simulink model "Final_EWASP_VC"  (R2022a)
settings: Solver=ode1  StartTime=0.0  StopTime=24*3600  FixedStep=10  RelTol=1e-3
values from neighbouring files (symbols this model uses):
  Aux_Threshold = 52    [Setup_Code_EWASP_VC.m]
  buildingAge = 2005    [Setup_Code_EWASP_VC.m]
  ceilingHeight = 2.4    [Setup_Code_EWASP_VC.m]
  conductiveHconnectMatrix = [ ... (first row only)    [Setup_Code_EWASP_VC.m]
  cRoofGreen = 100000    [Setup_Code_EWASP_VC.m]
  Defrost_After_Time = 30    [Setup_Code_EWASP_VC.m]
  DHWDemandProfile = occFreegainHotwaterElecTestPassiveOcc3(:,3)    [Setup_Code_EWASP_VC.m]
  Elec_Max = Elec_Max*(30/24.2)    [Setup_Code_EWASP_VC.m]
  Elec_Mid = Elec_Mid*(30/24.2)    [Setup_Code_EWASP_VC.m]
  Elec_Min = Elec_Min*(30/24.2)    [Setup_Code_EWASP_VC.m]
  ElecDemandProfile = occFreegainHotwaterElecTestPassiveOcc3(:,4)    [Setup_Code_EWASP_VC.m]
  ElecFixed = [Elec_Max(6,2) Elec_Max(6,4) Elec_Max(6,6) Elec_Max(6,7) ... (first row only)    [Setup_Code_EWASP_VC.m]
  floorOrCeilingArea = floorOrCeilingArea*1.15    [Setup_Code_EWASP_VC.m]
  forceCold = 0    [Setup_Code_EWASP_VC.m]
  freegain = occFreegainHotwaterElecTestPassiveOcc3(:,2)-max(occupancy)*25    [Setup_Code_EWASP_VC.m]
  furnitureModelOn = 1    [Setup_Code_EWASP_VC.m]
  Heat_Max = Heat_Max*(30/24.2)    [Setup_Code_EWASP_VC.m]
  Heat_Mid = Heat_Mid*(30/24.2)    [Setup_Code_EWASP_VC.m]
  Heat_Min = Heat_Min*(30/24.2)    [Setup_Code_EWASP_VC.m]
  HeatFixed = [Heat_Max(6,2) Heat_Max(6,4) Heat_Max(6,6) Heat_Max(6,7) ... (first row only)    [Setup_Code_EWASP_VC.m]
  HeatingOnProfile = repmat(HeatingOnProfile,365,1)    [Setup_Code_EWASP_VC.m]
  HEX_ReturnLowerLimit = 52.5    [Setup_Code_EWASP_VC.m]
  HEX_ReturnUpperLimit = 55    [Setup_Code_EWASP_VC.m]
  LeakMultiplier = 1+(2*(rand()-0.5)/10)    [Setup_Code_EWASP_VC.m]
  loopCap = 15    [Setup_Code_EWASP_VC.m]
  maxOcc = max(occupancyProfile)    [Setup_Code_EWASP_VC.m]
  NESW_wallArea = max(NESW_Lengths*ceilingHeight-NESW_Windows,0)    [Setup_Code_EWASP_VC.m]
  NESW_Windows = [ ... (first row only)    [Setup_Code_EWASP_VC.m]
  numRooms = roomCount    [Setup_Code_EWASP_VC.m]
  offsetDays = 0    [Setup_Code_EWASP_VC.m]
  pumpChoice = pumpChoices(MinIndex,1)    [Setup_Code_EWASP_VC.m]
  pumpRamp = 180    [Setup_Code_EWASP_VC.m]
  ReturnLowerLimit = 37.5    [Setup_Code_EWASP_VC.m]
  ReturnUpperLimit = 40    [Setup_Code_EWASP_VC.m]
  RoofIrradiance = Flat_NS_EW_RoofIrradiance(:,1)    [Setup_Code_EWASP_VC.m]
  roofStartTemp = ones(11,1)*20    [Setup_Code_EWASP_VC.m]
  rooftype = 0    [Setup_Code_EWASP_VC.m]
  RoomDataMatrix = [zeros(1,12);ones(1,12)*wallDensity;zeros(1,12);ones(1,12)*wallU;ones(1,12)*windowU;ones(1,12)*floorU;ones(1,12)*ceilingU;zeros(1,12);windowArea, 0;floorOrCeilingArea;zeros(1,12);floorOrCeilingArea*ceilingHeight]    [Setup_Code_EWASP_VC.m]
  roomVol = roomVol*1.15    [Setup_Code_EWASP_VC.m]
  slabStartTemp = (GroundTempTimeSeries(offsetDays*1440+1,1)+thermostatSetting)/2    [Setup_Code_EWASP_VC.m]
  SlackRequest = zeros(1440,1)    [Setup_Code_EWASP_VC.m]
  SolarThermalExists = 0    [Setup_Code_EWASP_VC.m]
  SourceFixed = HeatFixed-ElecFixed    [Setup_Code_EWASP_VC.m]
  StateSeries = StateSeriesGenerator(22,7,1)    [Setup_Code_EWASP_VC.m]
  Tank_Lower_Temp = 49.5    [Setup_Code_EWASP_VC.m]
  Tank_Upper_Temp = 52    [Setup_Code_EWASP_VC.m]
  Tank_Volume_m3 = 0.15    [Setup_Code_EWASP_VC.m]
  TankHeatHour = randi([1 5])-1    [Setup_Code_EWASP_VC.m]
  thermostatSetting = 20.0    (= 20)    [Setup_Code_EWASP_VC.m]
  upDown = [0;0;0;0;1;1;1;1;1;1;1]    [Setup_Code_EWASP_VC.m]
  variableASHP = 1    [Setup_Code_EWASP_VC.m]
  wallStartTempExt = thermostatSetting*(0.266+0.00215*outdoorStartTemp+0.018*wallU+0.00113*outdoorStartTemp*wallU+0.0068*wallU^2)    [Setup_Code_EWASP_VC.m]
undefined symbols (not defined in the file or in its folder): a, ceilingU, condUDMatrix, convUDMatrix, deltaPEXPANDED_E, deltaPEXPANDED_E2, deltaPEXPANDED_N, deltaPEXPANDED_N2, deltaPEXPANDED_S, deltaPEXPANDED_S2, deltaPEXPANDED_W, deltaPEXPANDED_W2, DesiredDHWTemp, DesiredFlowTempVsInOutDeltaTemp, DiffuseHorizontal, DiscIntNeverNeededParam, DNI, dwnAndConcrete, DWORK_A_HX, DWORK_CHK_FLU, DWORK_CP_NODE, DWORK_DH, DWORK_FLUID, DWORK_HCON, DWORK_LOSS, DWORK_MDOTDOWN, DWORK_MDOTIN, DWORK_MDOTUP, DWORK_MIX, DWORK_PRESS, DWORK_QDOTIN, DWORK_RHO_NODE, DWORK_TIN, DWORK_TS_OLD, DWORK_V_NODE, GroundTempTimeSeries, HCM, HCM2, HCM_closed, HCM_closed2, intermediateU, IsTop, massFlowMatrix, neighbourMatrix, numericalRoomUse, RadiatorMatrix, room2roomflowmatrix_E, room2roomflowmatrix_E2, room2roomflowmatrix_N, room2roomflowmatrix_N2, room2roomflowmatrix_S, room2roomflowmatrix_S2, room2roomflowmatrix_W, room2roomflowmatrix_W2, StateAirInEXPANDED_E, StateAirInEXPANDED_E2, StateAirInEXPANDED_N, StateAirInEXPANDED_N2, StateAirInEXPANDED_S, StateAirInEXPANDED_S2 ... (+23)
libraries: simulink x6, dspsigops x4, dspmtrx3 x4, carnot x3, spsEdgeDetectorLib x2, dspstat3 x2, powerlib_meascontrol x1, simulink_extras x1
(part 27 of 27)

== matlab function Final_EWASP_VC/Subsystem_Room8/Bedroom3/Subsystem4/MATLAB Function2 ==
  data: Angle_NEWS output; angleSeries input; NEWS_DNI output; DNISeries input; DiffSeries input; Time input; offsetDays input; NESW_Windows input; roomNumber input; NEWS_Diff output
function [Angle_NEWS,NEWS_DNI,NEWS_Diff] = SolarSeriesDataExtractor(angleSeries,DNISeries,DiffSeries,Time,offsetDays,NESW_Windows,roomNumber)

%deltaTexternalNEWS=zeros(1,4);

Angle_NEWS=angleSeries(ceil((offsetDays*1440)+Time/60+0.00001),1:4);
DNI=DNISeries(ceil((offsetDays*1440)+Time/60+0.00001),1);
Diff=DiffSeries(ceil((offsetDays*1440)+Time/60+0.00001),1);%extracts correct Diff per unit horizontal area for the timestep (corrected for wall tilt at a later stage

NEWS_windowArea=NESW_Windows;
NEWS_windowArea([3 4],:)=NEWS_windowArea([4 3],:);

RoomWindowAreas_NEWS=NEWS_windowArea(:,roomNumber)';


NEWS_DNI=RoomWindowAreas_NEWS*DNI;
NEWS_Diff=RoomWindowAreas_NEWS*Diff;

== matlab function Final_EWASP_VC/Subsystem_Room2/Kitchen/Subsystem1/MATLAB Function1 ==
  data: PU_AreaIrradianceTotal output; angleSeries input; NEWS_Irradiance output; DNISeries input; DiffSeries input; Time input; offsetDays input; SurfaceAlbedo input; NESW_wallArea input; roomNumber input; c_OutPU input; deltaTexternalNEWS output
function [PU_AreaIrradianceTotal, NEWS_Irradiance,deltaTexternalNEWS] = SolarSeriesToExtWallGains(angleSeries,DNISeries,DiffSeries,Time,offsetDays,SurfaceAlbedo,NESW_wallArea,roomNumber,c_OutPU)

%deltaTexternalNEWS=zeros(1,4);

Angle_NEWS=angleSeries(ceil((offsetDays*1440)+Time/60+0.00001),1:4);
DNI=DNISeries(ceil((offsetDays*1440)+Time/60+0.00001),1);

PU_AreaDiff=DiffSeries(ceil((offsetDays*1440)+Time/60+0.00001),1)/2;%extracts correct Diff for the timestep, factor of 1/2 corrects for 90 degree walls (so only half Diff irradiance can be utilised)
PU_AreaDNI=cos(deg2rad(Angle_NEWS))*DNI;
NEWS_wallArea=NESW_wallArea;
NEWS_wallArea([3 4],:)=NEWS_wallArea([4 3],:);

RoomWallAreas_NEWS=NEWS_wallArea(:,roomNumber)';
PU_AreaIrradianceTotal=(PU_AreaDNI+PU_AreaDiff)*(1-SurfaceAlbedo);

NEWS_Irradiance=RoomWallAreas_NEWS.*PU_AreaIrradianceTotal;
deltaTexternalNEWS=NEWS_Irradiance./(c_OutPU*RoomWallAreas_NEWS);

for i=1:4
   
    if RoomWallAreas_NEWS(1,i)==0
        deltaTexternalNEWS(1,i)=0;
    else
        
    end
    
end

== matlab function Final_EWASP_VC/Subsystem_Room5/Landing/Subsystem2/MATLAB Function1 ==
  data: PU_AreaIrradianceTotal output; angleSeries input; NEWS_Irradiance output; DNISeries input; DiffSeries input; Time input; offsetDays input; SurfaceAlbedo input; NESW_wallArea input; roomNumber input; c_OutPU input; deltaTexternalNEWS output
function [PU_AreaIrradianceTotal, NEWS_Irradiance,deltaTexternalNEWS] = SolarSeriesToExtWallGains(angleSeries,DNISeries,DiffSeries,Time,offsetDays,SurfaceAlbedo,NESW_wallArea,roomNumber,c_OutPU)

%deltaTexternalNEWS=zeros(1,4);

Angle_NEWS=angleSeries(ceil((offsetDays*1440)+Time/60+0.00001),1:4);
DNI=DNISeries(ceil((offsetDays*1440)+Time/60+0.00001),1);

PU_AreaDiff=DiffSeries(ceil((offsetDays*1440)+Time/60+0.00001),1)/2;%extracts correct Diff for the timestep, factor of 1/2 corrects for 90 degree walls (so only half Diff irradiance can be utilised)
PU_AreaDNI=cos(deg2rad(Angle_NEWS))*DNI;
NEWS_wallArea=NESW_wallArea;
NEWS_wallArea([3 4],:)=NEWS_wallArea([4 3],:);

RoomWallAreas_NEWS=NEWS_wallArea(:,roomNumber)';
PU_AreaIrradianceTotal=(PU_AreaDNI+PU_AreaDiff)*(1-SurfaceAlbedo);

NEWS_Irradiance=RoomWallAreas_NEWS.*PU_AreaIrradianceTotal;
deltaTexternalNEWS=NEWS_Irradiance./(c_OutPU*RoomWallAreas_NEWS);

for i=1:4
   
    if RoomWallAreas_NEWS(1,i)==0
        deltaTexternalNEWS(1,i)=0;
    else
        
    end
    
end

== matlab function Final_EWASP_VC/Subsystem_Room1/Lounge//Dining/Radiator w//Thermostatic Control2/MATLAB Function ==
  data: MassRad input; heatCapRad input; mdotRad input; Tflow input; Tnode1 input; Tnode2 input; deltaT1 output; deltaT2 output; nominalHeat input; nominalDeltaT input; Troom input; Qtoroom output
function [deltaT1,deltaT2,Qtoroom]=fcn(MassRad,heatCapRad, mdotRad, Tflow,Tnode1,Tnode2,nominalHeat,nominalDeltaT,Troom)


if  Tnode1 == Tnode2 || Tnode1 <= Troom || Tnode2 <= Troom %if lmtd methodnis problemtatic, use arithmetic method
    radiatorHeatOut=sign(((Tnode1+Tnode2) /2)-Troom)*abs((nominalHeat)*((((Tnode1+Tnode2) /2)-Troom)/nominalDeltaT)^1.3);
deltaT1=(mdotRad*4180*(Tflow-Tnode1))/((heatCapRad*MassRad)/2);
deltaT2=(mdotRad*4180*(Tnode1-Tnode2)-radiatorHeatOut)/((heatCapRad*MassRad)/2);

else 
  
   radiatorHeatOut=(nominalHeat/nominalDeltaT^1.3)*((Tnode1-Tnode2)/log((Tnode1-Troom)/(Tnode2-Troom)))^1.3;
   radiatorHeatOut=real(radiatorHeatOut);
deltaT1=(mdotRad*4180*(Tflow-Tnode1))/((heatCapRad*MassRad)/2);
deltaT2=(mdotRad*4180*(Tnode1-Tnode2)-radiatorHeatOut)/((heatCapRad*MassRad)/2);

   deltaT1=real(deltaT1);
   deltaT2=real(deltaT2);
    

end

Qtoroom=real(radiatorHeatOut);

== matlab function Final_EWASP_VC/Airflow Model/MATLAB Function ==
  data: WindSpeed input; WindIndex output; Tin_Avg input; T_out input; StackIndex output; WindDir input; DirIndex output
function [WindIndex,StackIndex,DirIndex] = fcn(WindSpeed,Tin_Avg,T_out,WindDir)

WindspeedLookUp=[0,1,2,3,5,8,12,15,18,21,25,30];
DeltaTemp=[0, 10, 20];

delT=(Tin_Avg-T_out);


[~,closestIndex] = min(abs(WindspeedLookUp-WindSpeed));
[~,closestIndex2] = min(abs(DeltaTemp-delT));

if WindDir == 1
    DirIndex=1;
elseif WindDir == 2
DirIndex=2;
elseif WindDir == 3
DirIndex=3;
elseif WindDir == 4
    DirIndex=4;
else
    error('wind direction must be either 1 (north) 2 (east) 3 (south) or 4 (west)')
end
WindIndex = closestIndex;
StackIndex = closestIndex2;

== matlab function Final_EWASP_VC/Airflow Model/MATLAB Function1 ==
  settings: updateMethod=DISCRETE  sampleTime=900
  data: WindSpeed input; WindIndex output; Tin_Avg input; T_out input; StackIndex output; WindDir input; DirIndex output
function [WindIndex,StackIndex,DirIndex] = fcn(WindSpeed,Tin_Avg,T_out,WindDir)

WindspeedLookUp=[0,1,2,3,5,8,12,15,18,21,25,30];
DeltaTemp=[0, 10, 20];

delT=(Tin_Avg-T_out);


[~,closestIndex] = min(abs(WindspeedLookUp-WindSpeed));
[~,closestIndex2] = min(abs(DeltaTemp-delT));

if WindDir == 1
    DirIndex=1;
elseif WindDir == 2
DirIndex=2;
elseif WindDir == 3
DirIndex=3;
elseif WindDir == 4
    DirIndex=4;
else
    error('wind direction must be either 1 (north) 2 (east) 3 (south) or 4 (west)')
end
WindIndex = closestIndex;
StackIndex = closestIndex2;

== matlab function Final_EWASP_VC/Airflow Model/StateLoader ==
  settings: updateMethod=DISCRETE  sampleTime=10
  data: R2R_out output size=[11 11]; windIndex input; stackIndex input; windDir input; room2roomflowmatrix_N input; room2roomflowmatrix_E input; room2roomflowmatrix_S input; room2roomflowmatrix_W input; StateAirInEXPANDED_N input; StateAirInEXPANDED_E input; StateAirInEXPANDED_S input; StateAirInEXPANDED_W input; StateAirOutEXPANDED_N input; StateAirOutEXPANDED_E input; StateAirOutEXPANDED_S input; StateAirOutEXPANDED_W input; deltaPEXPANDED_N input; deltaPEXPANDED_E input; deltaPEXPANDED_S input; deltaPEXPANDED_W input; numRooms input; StateAirIn_out output size=[11 1]; StateAirOut_out output size=[11 1]; deltaP output
function [R2R_out, StateAirIn_out,StateAirOut_out,deltaP] = fcn(windIndex,stackIndex,windDir,room2roomflowmatrix_N,room2roomflowmatrix_E,room2roomflowmatrix_S,room2roomflowmatrix_W,StateAirInEXPANDED_N,StateAirInEXPANDED_E,StateAirInEXPANDED_S,StateAirInEXPANDED_W,StateAirOutEXPANDED_N,StateAirOutEXPANDED_E,StateAirOutEXPANDED_S,StateAirOutEXPANDED_W,deltaPEXPANDED_N,deltaPEXPANDED_E,deltaPEXPANDED_S,deltaPEXPANDED_W,numRooms)

if windDir == 1
    
R2R_out=room2roomflowmatrix_N((windIndex-1)*numRooms+1:windIndex*numRooms,(stackIndex-1)*numRooms+1:stackIndex*numRooms);
StateAirIn_out=StateAirInEXPANDED_N((windIndex-1)*numRooms+1:windIndex*numRooms,stackIndex);
StateAirOut_out=StateAirOutEXPANDED_N((windIndex-1)*numRooms+1:windIndex*numRooms,stackIndex);
deltaP=deltaPEXPANDED_N(windIndex,stackIndex);

elseif windDir == 2
    
    R2R_out=room2roomflowmatrix_E((windIndex-1)*numRooms+1:windIndex*numRooms,(stackIndex-1)*numRooms+1:stackIndex*numRooms);
StateAirIn_out=StateAirInEXPANDED_E((windIndex-1)*numRooms+1:windIndex*numRooms,stackIndex);
StateAirOut_out=StateAirOutEXPANDED_E((windIndex-1)*numRooms+1:windIndex*numRooms,stackIndex);
deltaP=deltaPEXPANDED_E(windIndex,stackIndex);
    
elseif windDir == 3
        
    R2R_out=room2roomflowmatrix_S((windIndex-1)*numRooms+1:windIndex*numRooms,(stackIndex-1)*numRooms+1:stackIndex*numRooms);
StateAirIn_out=StateAirInEXPANDED_S((windIndex-1)*numRooms+1:windIndex*numRooms,stackIndex);
StateAirOut_out=StateAirOutEXPANDED_S((windIndex-1)*numRooms+1:windIndex*numRooms,stackIndex);
deltaP=deltaPEXPANDED_S(windIndex,stackIndex);
    
elseif windDir == 4
            
    R2R_out=room2roomflowmatrix_W((windIndex-1)*numRooms+1:windIndex*numRooms,(stackIndex-1)*numRooms+1:stackIndex*numRooms);
StateAirIn_out=StateAirInEXPANDED_W((windIndex-1)*numRooms+1:windIndex*numRooms,stackIndex);
StateAirOut_out=StateAirOutEXPANDED_W((windIndex-1)*numRooms+1:windIndex*numRooms,stackIndex);
deltaP=deltaPEXPANDED_W(windIndex,stackIndex);
    
else
  error('windDir must equal 1,2,3, or 4')          
end

%R2R_out=R2R_out+zeros(11,11);
%R2R_out=R2R_out(11,11);
%StateAirIn_out=StateAirIn_out+zeros(11,1);
%StateAirOut_out=StateAirOut_out+zeros(11,1);

== matlab function Final_EWASP_VC/Airflow Model/StateLoader1 ==
  settings: updateMethod=DISCRETE  sampleTime=10
  data: windIndex input; stackIndex input; windDir input; room2roomflowmatrix_N input; room2roomflowmatrix_E input; room2roomflowmatrix_S input; room2roomflowmatrix_W input; StateAirInEXPANDED_N input; StateAirInEXPANDED_E input; StateAirInEXPANDED_S input; StateAirInEXPANDED_W input; StateAirOutEXPANDED_N input; StateAirOutEXPANDED_E input; StateAirOutEXPANDED_S input; StateAirOutEXPANDED_W input; deltaPEXPANDED_N input; deltaPEXPANDED_E input; deltaPEXPANDED_S input; deltaPEXPANDED_W input; numRooms input; R2R_out output size=[11 11]; StateAirIn_out output size=[11 1]; StateAirOut_out output size=[11 1]; deltaP output
function [R2R_out,StateAirIn_out,StateAirOut_out,deltaP] = fcn(windIndex,stackIndex,windDir,room2roomflowmatrix_N,room2roomflowmatrix_E,room2roomflowmatrix_S,room2roomflowmatrix_W,StateAirInEXPANDED_N,StateAirInEXPANDED_E,StateAirInEXPANDED_S,StateAirInEXPANDED_W,StateAirOutEXPANDED_N,StateAirOutEXPANDED_E,StateAirOutEXPANDED_S,StateAirOutEXPANDED_W,deltaPEXPANDED_N,deltaPEXPANDED_E,deltaPEXPANDED_S,deltaPEXPANDED_W,numRooms)

if windDir == 1
    
R2R_out=room2roomflowmatrix_N((windIndex-1)*numRooms+1:windIndex*numRooms,(stackIndex-1)*numRooms+1:stackIndex*numRooms);
StateAirIn_out=StateAirInEXPANDED_N((windIndex-1)*numRooms+1:windIndex*numRooms,stackIndex);
StateAirOut_out=StateAirOutEXPANDED_N((windIndex-1)*numRooms+1:windIndex*numRooms,stackIndex);
deltaP=deltaPEXPANDED_N(windIndex,stackIndex);

elseif windDir == 2
    
    R2R_out=room2roomflowmatrix_E((windIndex-1)*numRooms+1:windIndex*numRooms,(stackIndex-1)*numRooms+1:stackIndex*numRooms);
StateAirIn_out=StateAirInEXPANDED_E((windIndex-1)*numRooms+1:windIndex*numRooms,stackIndex);
StateAirOut_out=StateAirOutEXPANDED_E((windIndex-1)*numRooms+1:windIndex*numRooms,stackIndex);
deltaP=deltaPEXPANDED_E(windIndex,stackIndex);
    
elseif windDir == 3
        
    R2R_out=room2roomflowmatrix_S((windIndex-1)*numRooms+1:windIndex*numRooms,(stackIndex-1)*numRooms+1:stackIndex*numRooms);
StateAirIn_out=StateAirInEXPANDED_S((windIndex-1)*numRooms+1:windIndex*numRooms,stackIndex);
StateAirOut_out=StateAirOutEXPANDED_S((windIndex-1)*numRooms+1:windIndex*numRooms,stackIndex);
deltaP=deltaPEXPANDED_S(windIndex,stackIndex);
    
elseif windDir == 4
            
    R2R_out=room2roomflowmatrix_W((windIndex-1)*numRooms+1:windIndex*numRooms,(stackIndex-1)*numRooms+1:stackIndex*numRooms);
StateAirIn_out=StateAirInEXPANDED_W((windIndex-1)*numRooms+1:windIndex*numRooms,stackIndex);
StateAirOut_out=StateAirOutEXPANDED_W((windIndex-1)*numRooms+1:windIndex*numRooms,stackIndex);
deltaP=deltaPEXPANDED_W(windIndex,stackIndex);
    
else
  error('windDir must equal 1,2,3, or 4')          
end

%R2R_out=R2R_out+zeros(11,11);
%StateAirIn_out=StateAirIn_out+zeros(11,1);
%StateAirOut_out=StateAirOut_out+zeros(11,1);

== matlab function Final_EWASP_VC/Airflow Model/Subsystem1/Subsystem/Actual buoyancy ==
  data: u input; y output; v input; w input
function y  = fcn(u,v,w)

y = w.*(1-u./v);

== matlab function Final_EWASP_VC/Airflow Model/Subsystem1/Subsystem/Remove nan values ==
  data: y output; u input
function y  = fcn(u)

u(isnan(u))=0;
y=u;

== matlab function Final_EWASP_VC/Airflow Model/Subsystem1/Subsystem/Subsystem1/Temp2density ==
  data: u input; y output
function y  = fcn(u)

y = -0.0042*u+1.2898;

== matlab function Final_EWASP_VC/Airflow Model/Subsystem1/Subsystem/Subsystem1/Temp2density1 ==
  data: u input; y output
function y  = fcn(u)

y = -0.0042*u+1.2898;

== matlab function Final_EWASP_VC/Airflow Model/Subsystem1/Subsystem/Subsystem1/Temp2density2 ==
  data: u input; y output
function y  = fcn(u)

y = -0.0042*u+1.2898;

== matlab function Final_EWASP_VC/Airflow Model/Subsystem1/Subsystem/Subsystem1/floorDensityCorrection ==
  data: u input; y output; v input; w input
function y  = fcn(u,v,w)

a=u-u.*2.718^((-9.80665*0.0289644*2.7)/(8.31446*(w+273.15)));


y=repmat(v,1,length(v))*a;

== matlab function Final_EWASP_VC/Airflow Model/Subsystem1/Subsystem/Subsystem1/tempVector to average ==
  data: u input; y output
function y = fcn(u)

y = mean(u);

== matlab function Final_EWASP_VC/Subsystem_Room1/Lounge//Dining/Subsystem1/MATLAB Function ==
  data: uValWall input; deltaTint output; c_InPU input; c_MidPU input; c_OutPU input; T_InWallNEWS input; T_MidWallNEWS input; T_OutWallNEWS input; T_Room input; T_AmbientSeries input; windSpeedSeries input; deltaTmid output; deltaTout output; NESW_wallArea input; roomNumber input; logRoomHeatLoss output; Time input; offsetDays input
function [deltaTint,deltaTmid,deltaTout,logRoomHeatLoss] = fcn(uValWall,c_InPU,c_MidPU,c_OutPU,T_InWallNEWS, T_MidWallNEWS,T_OutWallNEWS,T_Room,T_AmbientSeries,windSpeedSeries,NESW_wallArea,roomNumber,Time,offsetDays)




  deltaTint=zeros(1,4);
   deltaTmid=zeros(1,4);
    deltaTout=zeros(1,4);
    logRoomHeatLoss=zeros(1,4);

    v_Wind=windSpeedSeries(ceil((offsetDays*1440)+Time/60+0.00001),1);
   T_Ambient=T_AmbientSeries(ceil((offsetDays*1440)+Time/60+0.00001),1);
    
k_InMid=uValWall*2;
k_OutMid=uValWall*2;


NEWS_wallArea=NESW_wallArea;
NEWS_wallArea([3 4],:)=NEWS_wallArea([4 3],:);
RoomWallAreas_NEWS=NEWS_wallArea(:,roomNumber)';


for i=1:4
    
    if RoomWallAreas_NEWS(1,i)>0

c_In=c_InPU*RoomWallAreas_NEWS(1,i);
c_Mid=c_MidPU*RoomWallAreas_NEWS(1,i);
c_Out=c_OutPU*RoomWallAreas_NEWS(1,i);

T_InWall=T_InWallNEWS(1,i);
T_MidWall=T_MidWallNEWS(1,i);
T_OutWall=T_OutWallNEWS(1,i);
    
aA=[-(k_InMid*RoomWallAreas_NEWS(1,i))/c_In (k_InMid*RoomWallAreas_NEWS(1,i))/c_In 0
 (k_InMid*RoomWallAreas_NEWS(1,i))/c_Mid -((k_InMid+k_OutMid)*RoomWallAreas_NEWS(1,i))/c_Mid (k_OutMid*RoomWallAreas_NEWS(1,i))/c_Mid
 0 (k_OutMid*RoomWallAreas_NEWS(1,i))/c_Out -(k_OutMid*RoomWallAreas_NEWS(1,i))/c_Out];

bA=[1/c_In 0 0
 0 1/c_Mid 0
 0 0 1/c_Out];
    
ab=[T_InWall
    T_MidWall
    T_OutWall];

bb=[(2.5*(T_Room-T_InWall)+5.6*(T_Room-T_InWall))*RoomWallAreas_NEWS(1,i)
0    
(2.8+3*v_Wind)*(T_Ambient-T_OutWall)+5.6*(T_Ambient-T_OutWall)*RoomWallAreas_NEWS(1,i)];

deltaT=aA*ab+bA*bb;

    deltaTint(1,i)=deltaT(1,1);
   deltaTmid(1,i)=deltaT(2,1);
    deltaTout(1,i)=deltaT(3,1);
    
    logRoomHeatLoss(1,i)=bb(1,1);
    
    else
        
        deltaTint(1,i)=0;
   deltaTmid(1,i)=0;
    deltaTout(1,i)=0;
        
    logRoomHeatLoss(1,i)=0;
    
    end
    
end

== matlab function Final_EWASP_VC/Airflow Model/Subsystem1/Subsystem/Subsystem1/tempVector to matrices ==
  data: u input; y output; x output
function [y,x] = fcn(u)

y = repmat(u,1,size(u,1));
x=y';

== matlab function Final_EWASP_VC/Airflow Model/Subsystem1/Subsystem/max buoyancy ==
  data: u input; y output; v input
function y  = fcn(u,v)

y = (u*0.055).*abs(9.81*v.*ones(size(u,1),size(u,1))./u).^0.5;

== matlab function Final_EWASP_VC/Airflow Model/Subsystem1/Subsystem/pflood ==
  data: u input; y output
function y  = fcn(u)

y = ((1/0.3)*0.942^2*9.81*u*1)/(2*1);

== matlab function Final_EWASP_VC/Airflow Model/Subsystem1/Subsystem/tempVector to matrices ==
  data: u input; y output; x output
function [y,x] = fcn(u)

a=u;
y = repmat(a,1,length(a));
x=y';

== matlab function Final_EWASP_VC/Airflow Model/Subsystem2/Subsystem/Actual buoyancy ==
  data: u input; y output; v input; w input
function y  = fcn(u,v,w)

y = w.*(1-u./v);

== matlab function Final_EWASP_VC/Airflow Model/Subsystem2/Subsystem/Remove nan values ==
  data: y output; u input
function y  = fcn(u)

u(isnan(u))=0;
y=u;

== matlab function Final_EWASP_VC/Airflow Model/Subsystem2/Subsystem/Subsystem1/Temp2density ==
  data: u input; y output
function y  = fcn(u)

y = -0.0042*u+1.2898;

== matlab function Final_EWASP_VC/Airflow Model/Subsystem2/Subsystem/Subsystem1/Temp2density1 ==
  data: u input; y output
function y  = fcn(u)

y = -0.0042*u+1.2898;

== matlab function Final_EWASP_VC/Airflow Model/Subsystem2/Subsystem/Subsystem1/Temp2density2 ==
  data: u input; y output
function y  = fcn(u)

y = -0.0042*u+1.2898;

== matlab function Final_EWASP_VC/Airflow Model/Subsystem2/Subsystem/Subsystem1/floorDensityCorrection ==
  data: u input; y output; v input; w input
function y  = fcn(u,v,w)

a=u-u.*2.718^((-9.80665*0.0289644*2.7)/(8.31446*(w+273.15)));


y=repmat(v,1,length(v))*a;

== matlab function Final_EWASP_VC/Airflow Model/Subsystem2/Subsystem/Subsystem1/tempVector to average ==
  data: u input; y output
function y = fcn(u)

y = mean(u);

== matlab function Final_EWASP_VC/Airflow Model/Subsystem2/Subsystem/Subsystem1/tempVector to matrices ==
  data: u input; y output; x output
function [y,x] = fcn(u)

y = repmat(u,1,size(u,1));
x=y';

== matlab function Final_EWASP_VC/Airflow Model/Subsystem2/Subsystem/max buoyancy ==
  data: u input; y output; v input
function y  = fcn(u,v)

y = (u*0.055).*abs(9.81*v.*ones(size(u,1),size(u,1))./u).^0.5;

== matlab function Final_EWASP_VC/Airflow Model/Subsystem2/Subsystem/pflood ==
  data: u input; y output
function y  = fcn(u)

y = ((1/0.3)*0.942^2*9.81*u*1)/(2*1);

== matlab function Final_EWASP_VC/Airflow Model/Subsystem2/Subsystem/tempVector to matrices ==
  data: u input; y output; x output
function [y,x] = fcn(u)

a=u;
y = repmat(a,1,length(a));
x=y';

== matlab function Final_EWASP_VC/Subsystem_Room1/Lounge//Dining/Subsystem3/MATLAB Function ==
  data: uValWall input; deltaTint output; c_InPU input; c_MidPU input; c_OutPU input; T_InWall input; T_MidWall input; T_OutWall input; T_Room input; T_AmbientSeries input; windSpeedSeries input; deltaTmid output; deltaTout output; ceilArea input; roomNumber input; logRoomHeatLoss output; Time input; offsetDays input
function [deltaTint,deltaTmid,deltaTout,logRoomHeatLoss] = fcn(uValWall,c_InPU,c_MidPU,c_OutPU,T_InWall, T_MidWall,T_OutWall,T_Room,T_AmbientSeries,windSpeedSeries,ceilArea,roomNumber,Time,offsetDays)




  deltaTint=zeros(1,1);
   deltaTmid=zeros(1,1);
    deltaTout=zeros(1,1);
    logRoomHeatLoss=zeros(1,1);

    v_Wind=windSpeedSeries(ceil((offsetDays*1440)+Time/60+0.00001),1);
   T_Ambient=T_AmbientSeries(ceil((offsetDays*1440)+Time/60+0.00001),1);
    
k_InMid=uValWall*2;
k_OutMid=uValWall*2;




    
    if ceilArea>0

c_In=c_InPU*ceilArea;
c_Mid=c_MidPU*ceilArea;
c_Out=c_OutPU*ceilArea;

    
aA=[-(k_InMid*ceilArea)/c_In (k_InMid*ceilArea)/c_In 0
 (k_InMid*ceilArea)/c_Mid -((k_InMid+k_OutMid)*ceilArea)/c_Mid (k_OutMid*ceilArea)/c_Mid
 0 (k_OutMid*ceilArea)/c_Out -(k_OutMid*ceilArea)/c_Out];

bA=[1/c_In 0 0
 0 1/c_Mid 0
 0 0 1/c_Out];
    
ab=[T_InWall
    T_MidWall
    T_OutWall];

bb=[(2.5*(T_Room-T_InWall)+5.6*(T_Room-T_InWall))*ceilArea
0    
(2.8+3*v_Wind)*(T_Ambient-T_OutWall)+5.6*(T_Ambient-T_OutWall)*ceilArea];

deltaT=aA*ab+bA*bb;

    deltaTint=deltaT(1,1);
   deltaTmid=deltaT(2,1);
    deltaTout=deltaT(3,1);
    
    logRoomHeatLoss=bb(1,1);
    
    else
        
        deltaTint=0;
   deltaTmid=0;
    deltaTout=0;
        
    logRoomHeatLoss=0;
    
    end

== matlab function Final_EWASP_VC/Subsystem_Room7/Bedroom 2/Subsystem3/MATLAB Function ==
  data: uValWall input; deltaTint output; c_InPU input; c_MidPU input; c_OutPU input; T_InWallNEWS input; T_MidWallNEWS input; T_OutWallNEWS input; T_Room input; T_AmbientSeries input; windSpeedSeries input; deltaTmid output; deltaTout output; NESW_wallArea input; roomNumber input; logRoomHeatLoss output; Time input; offsetDays input
function [deltaTint,deltaTmid,deltaTout,logRoomHeatLoss] = fcn(uValWall,c_InPU,c_MidPU,c_OutPU,T_InWallNEWS, T_MidWallNEWS,T_OutWallNEWS,T_Room,T_AmbientSeries,windSpeedSeries,NESW_wallArea,roomNumber,Time,offsetDays)




  deltaTint=zeros(1,4);
   deltaTmid=zeros(1,4);
    deltaTout=zeros(1,4);
    logRoomHeatLoss=zeros(1,4);

    v_Wind=windSpeedSeries(ceil((offsetDays*1440)+Time/60+0.00001),1);
   T_Ambient=T_AmbientSeries(ceil((offsetDays*1440)+Time/60+0.00001),1);
    
k_InMid=uValWall*2;
k_OutMid=uValWall*2;


NEWS_wallArea=NESW_wallArea;
NEWS_wallArea([3 4],:)=NEWS_wallArea([4 3],:);
RoomWallAreas_NEWS=NEWS_wallArea(:,roomNumber)';


for i=1:4
    
    if RoomWallAreas_NEWS(1,i)>0

c_In=c_InPU*RoomWallAreas_NEWS(1,i);
c_Mid=c_MidPU*RoomWallAreas_NEWS(1,i);
c_Out=c_OutPU*RoomWallAreas_NEWS(1,i);

T_InWall=T_InWallNEWS(1,i);
T_MidWall=T_MidWallNEWS(1,i);
T_OutWall=T_OutWallNEWS(1,i);
    
aA=[-(k_InMid*RoomWallAreas_NEWS(1,i))/c_In (k_InMid*RoomWallAreas_NEWS(1,i))/c_In 0
 (k_InMid*RoomWallAreas_NEWS(1,i))/c_Mid -((k_InMid+k_OutMid)*RoomWallAreas_NEWS(1,i))/c_Mid (k_OutMid*RoomWallAreas_NEWS(1,i))/c_Mid
 0 (k_OutMid*RoomWallAreas_NEWS(1,i))/c_Out -(k_OutMid*RoomWallAreas_NEWS(1,i))/c_Out];

bA=[1/c_In 0 0
 0 1/c_Mid 0
 0 0 1/c_Out];
    
ab=[T_InWall
    T_MidWall
    T_OutWall];

bb=[(2.5*(T_Room-T_InWall)+5.6*(T_Room-T_InWall))*RoomWallAreas_NEWS(1,i)
0    
(2.8+3*v_Wind)*(T_Ambient-T_OutWall)+5.6*(T_Ambient-T_OutWall)*RoomWallAreas_NEWS(1,i)];

deltaT=aA*ab+bA*bb;

    deltaTint(1,i)=deltaT(1,1);
   deltaTmid(1,i)=deltaT(2,1);
    deltaTout(1,i)=deltaT(3,1);
    
    logRoomHeatLoss(1,i)=bb(1,1);
    
    else
        
        deltaTint(1,i)=0;
   deltaTmid(1,i)=0;
    deltaTout(1,i)=0;
        
    logRoomHeatLoss(1,i)=0;
    
    end
    
end

== matlab function Final_EWASP_VC/Subsystem_Room7/Bedroom 2/Subsystem3/MATLAB Function1 ==
  data: PU_AreaIrradianceTotal output; angleSeries input; NEWS_Irradiance output; DNISeries input; DiffSeries input; Time input; offsetDays input; SurfaceAlbedo input; NESW_wallArea input; roomNumber input; c_OutPU input; deltaTexternalNEWS output
function [PU_AreaIrradianceTotal, NEWS_Irradiance,deltaTexternalNEWS] = SolarSeriesToExtWallGains(angleSeries,DNISeries,DiffSeries,Time,offsetDays,SurfaceAlbedo,NESW_wallArea,roomNumber,c_OutPU)

%deltaTexternalNEWS=zeros(1,4);

Angle_NEWS=angleSeries(ceil((offsetDays*1440)+Time/60+0.00001),1:4);
DNI=DNISeries(ceil((offsetDays*1440)+Time/60+0.00001),1);

PU_AreaDiff=DiffSeries(ceil((offsetDays*1440)+Time/60+0.00001),1)/2;%extracts correct Diff for the timestep, factor of 1/2 corrects for 90 degree walls (so only half Diff irradiance can be utilised)
PU_AreaDNI=cos(deg2rad(Angle_NEWS))*DNI;
NEWS_wallArea=NESW_wallArea;
NEWS_wallArea([3 4],:)=NEWS_wallArea([4 3],:);

RoomWallAreas_NEWS=NEWS_wallArea(:,roomNumber)';
PU_AreaIrradianceTotal=(PU_AreaDNI+PU_AreaDiff)*(1-SurfaceAlbedo);

NEWS_Irradiance=RoomWallAreas_NEWS.*PU_AreaIrradianceTotal;
deltaTexternalNEWS=NEWS_Irradiance./(c_OutPU*RoomWallAreas_NEWS);

for i=1:4
   
    if RoomWallAreas_NEWS(1,i)==0
        deltaTexternalNEWS(1,i)=0;
    else
        
    end
    
end

== matlab function Final_EWASP_VC/Subsystem_Room1/Lounge//Dining/Subsystem3/MATLAB Function1 ==
  data: Time input; offsetDays input; SurfaceAlbedo input; Tot_Irradiance output; RoofArea input; c_OutRoof input; deltaTexternal output; RoofIrradiance input
function [Tot_Irradiance, deltaTexternal] = SolarSeriesToExtWallGains(Time,offsetDays,SurfaceAlbedo,RoofArea,c_OutRoof,RoofIrradiance)

PU_AreaIrr=RoofIrradiance(ceil((offsetDays*1440)+Time/60+0.00001),1)/2;%extracts correct Diff for the timestep, factor of 1/2 corrects for 90 degree walls (so only half Diff irradiance can be utilised)


Tot_Irradiance=(RoofArea*PU_AreaIrr)*(1-SurfaceAlbedo);
deltaTexternal=Tot_Irradiance./(c_OutRoof*RoofArea);

    
end

== matlab function Final_EWASP_VC/Subsystem_Room6/Bedroom1/Subsystem3/MATLAB Function ==
  data: uValWall input; deltaTint output; c_InPU input; c_MidPU input; c_OutPU input; T_InWall input; T_MidWall input; T_OutWall input; T_Room input; T_AmbientSeries input; windSpeedSeries input; deltaTmid output; deltaTout output; ceilArea input; roomNumber input; logRoomHeatLoss output; Time input; offsetDays input
function [deltaTint,deltaTmid,deltaTout,logRoomHeatLoss] = fcn(uValWall,c_InPU,c_MidPU,c_OutPU,T_InWall, T_MidWall,T_OutWall,T_Room,T_AmbientSeries,windSpeedSeries,ceilArea,roomNumber,Time,offsetDays)




  deltaTint=zeros(1,1);
   deltaTmid=zeros(1,1);
    deltaTout=zeros(1,1);
    logRoomHeatLoss=zeros(1,1);

    v_Wind=windSpeedSeries(ceil((offsetDays*1440)+Time/60+0.00001),1);
   T_Ambient=T_AmbientSeries(ceil((offsetDays*1440)+Time/60+0.00001),1);
    
k_InMid=uValWall*2;
k_OutMid=uValWall*2;




    
    if ceilArea>0

c_In=c_InPU*ceilArea;
c_Mid=c_MidPU*ceilArea;
c_Out=c_OutPU*ceilArea;

    
aA=[-(k_InMid*ceilArea)/c_In (k_InMid*ceilArea)/c_In 0
 (k_InMid*ceilArea)/c_Mid -((k_InMid+k_OutMid)*ceilArea)/c_Mid (k_OutMid*ceilArea)/c_Mid
 0 (k_OutMid*ceilArea)/c_Out -(k_OutMid*ceilArea)/c_Out];

bA=[1/c_In 0 0
 0 1/c_Mid 0
 0 0 1/c_Out];
    
ab=[T_InWall
    T_MidWall
    T_OutWall];

bb=[(2.5*(T_Room-T_InWall)+5.6*(T_Room-T_InWall))*ceilArea
0    
(2.8+3*v_Wind)*(T_Ambient-T_OutWall)+5.6*(T_Ambient-T_OutWall)*ceilArea];

deltaT=aA*ab+bA*bb;

    deltaTint=deltaT(1,1);
   deltaTmid=deltaT(2,1);
    deltaTout=deltaT(3,1);
    
    logRoomHeatLoss=bb(1,1);
    
    else
        
        deltaTint=0;
   deltaTmid=0;
    deltaTout=0;
        
    logRoomHeatLoss=0;
    
    end

== matlab function Final_EWASP_VC/Subsystem_Room6/Bedroom1/Subsystem3/MATLAB Function1 ==
  data: Time input; offsetDays input; SurfaceAlbedo input; Tot_Irradiance output; RoofArea input; c_OutRoof input; deltaTexternal output; RoofIrradiance input
function [Tot_Irradiance, deltaTexternal] = SolarSeriesToExtWallGains(Time,offsetDays,SurfaceAlbedo,RoofArea,c_OutRoof,RoofIrradiance)

PU_AreaIrr=RoofIrradiance(ceil((offsetDays*1440)+Time/60+0.00001),1)/2;%extracts correct Diff for the timestep, factor of 1/2 corrects for 90 degree walls (so only half Diff irradiance can be utilised)


Tot_Irradiance=(RoofArea*PU_AreaIrr)*(1-SurfaceAlbedo);
deltaTexternal=Tot_Irradiance./(c_OutRoof*RoofArea);

    
end

== matlab function Final_EWASP_VC/Subsystem_Room2/Kitchen/Subsystem3/MATLAB Function ==
  data: uValWall input; deltaTint output; c_InPU input; c_MidPU input; c_OutPU input; T_InWall input; T_MidWall input; T_OutWall input; T_Room input; T_AmbientSeries input; windSpeedSeries input; deltaTmid output; deltaTout output; ceilArea input; roomNumber input; logRoomHeatLoss output; Time input; offsetDays input
function [deltaTint,deltaTmid,deltaTout,logRoomHeatLoss] = fcn(uValWall,c_InPU,c_MidPU,c_OutPU,T_InWall, T_MidWall,T_OutWall,T_Room,T_AmbientSeries,windSpeedSeries,ceilArea,roomNumber,Time,offsetDays)




  deltaTint=zeros(1,1);
   deltaTmid=zeros(1,1);
    deltaTout=zeros(1,1);
    logRoomHeatLoss=zeros(1,1);

    v_Wind=windSpeedSeries(ceil((offsetDays*1440)+Time/60+0.00001),1);
   T_Ambient=T_AmbientSeries(ceil((offsetDays*1440)+Time/60+0.00001),1);
    
k_InMid=uValWall*2;
k_OutMid=uValWall*2;




    
    if ceilArea>0

c_In=c_InPU*ceilArea;
c_Mid=c_MidPU*ceilArea;
c_Out=c_OutPU*ceilArea;

    
aA=[-(k_InMid*ceilArea)/c_In (k_InMid*ceilArea)/c_In 0
 (k_InMid*ceilArea)/c_Mid -((k_InMid+k_OutMid)*ceilArea)/c_Mid (k_OutMid*ceilArea)/c_Mid
 0 (k_OutMid*ceilArea)/c_Out -(k_OutMid*ceilArea)/c_Out];

bA=[1/c_In 0 0
 0 1/c_Mid 0
 0 0 1/c_Out];
    
ab=[T_InWall
    T_MidWall
    T_OutWall];

bb=[(2.5*(T_Room-T_InWall)+5.6*(T_Room-T_InWall))*ceilArea
0    
(2.8+3*v_Wind)*(T_Ambient-T_OutWall)+5.6*(T_Ambient-T_OutWall)*ceilArea];

deltaT=aA*ab+bA*bb;

    deltaTint=deltaT(1,1);
   deltaTmid=deltaT(2,1);
    deltaTout=deltaT(3,1);
    
    logRoomHeatLoss=bb(1,1);
    
    else
        
        deltaTint=0;
   deltaTmid=0;
    deltaTout=0;
        
    logRoomHeatLoss=0;
    
    end

== matlab function Final_EWASP_VC/Subsystem_Room1/Lounge//Dining/Subsystem1/MATLAB Function1 ==
  data: PU_AreaIrradianceTotal output; angleSeries input; NEWS_Irradiance output; DNISeries input; DiffSeries input; Time input; offsetDays input; SurfaceAlbedo input; NESW_wallArea input; roomNumber input; c_OutPU input; deltaTexternalNEWS output
function [PU_AreaIrradianceTotal, NEWS_Irradiance,deltaTexternalNEWS] = SolarSeriesToExtWallGains(angleSeries,DNISeries,DiffSeries,Time,offsetDays,SurfaceAlbedo,NESW_wallArea,roomNumber,c_OutPU)

%deltaTexternalNEWS=zeros(1,4);

Angle_NEWS=angleSeries(ceil((offsetDays*1440)+Time/60+0.00001),1:4);
DNI=DNISeries(ceil((offsetDays*1440)+Time/60+0.00001),1);

PU_AreaDiff=DiffSeries(ceil((offsetDays*1440)+Time/60+0.00001),1)/2;%extracts correct Diff for the timestep, factor of 1/2 corrects for 90 degree walls (so only half Diff irradiance can be utilised)
PU_AreaDNI=cos(deg2rad(Angle_NEWS))*DNI;
NEWS_wallArea=NESW_wallArea;
NEWS_wallArea([3 4],:)=NEWS_wallArea([4 3],:);

RoomWallAreas_NEWS=NEWS_wallArea(:,roomNumber)';
PU_AreaIrradianceTotal=(PU_AreaDNI+PU_AreaDiff)*(1-SurfaceAlbedo);

NEWS_Irradiance=RoomWallAreas_NEWS.*PU_AreaIrradianceTotal;
deltaTexternalNEWS=NEWS_Irradiance./(c_OutPU*RoomWallAreas_NEWS);

for i=1:4
   
    if RoomWallAreas_NEWS(1,i)==0
        deltaTexternalNEWS(1,i)=0;
    else
        
    end
    
end
